simulink model "CSK_Std_PulseTrain"  (R2014b)
settings: Solver=ode23s  StartTime=0.0  StopTime=150  RelTol=1e-12
undefined symbols (not defined in the file or in its folder): Rho, Sigma, x01, x02, x03
settings Model: Creator=Dan  LastModifiedBy=Dan

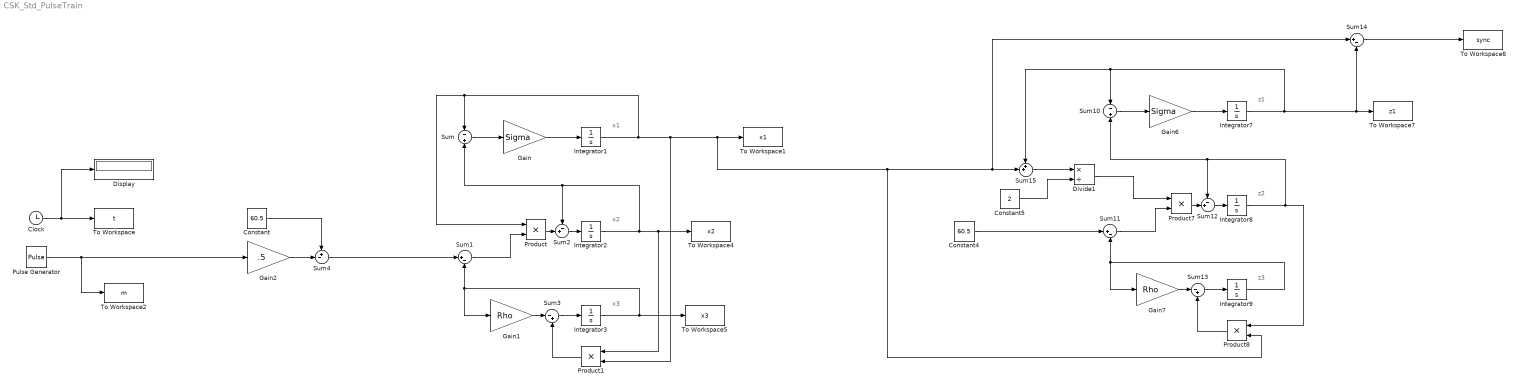
== system CSK_Std_PulseTrain ==
  note: x1
  note: x2
  note: x3
  note: z1
  note: z2
  note: z3
  Clock : Clock
  Constant : Constant  Value=60.5
  Constant4 : Constant  Value=60.5
  Constant5 : Constant  Value=2
  Display : Display
      settings: Decimation=5
  Divide1 : Product  Inputs=*/
  Gain : Gain  Gain=Sigma
  Gain1 : Gain  Gain=Rho
  Gain2 : Gain  Gain=.5
  Gain6 : Gain  Gain=Sigma
  Gain7 : Gain  Gain=Rho
  Integrator1 : Integrator  InitialCondition=x01
  Integrator2 : Integrator  InitialCondition=x02
  Integrator3 : Integrator  InitialCondition=x03
  Integrator7 : Integrator  InitialCondition=x01
  Integrator8 : Integrator  InitialCondition=x02
  Integrator9 : Integrator  InitialCondition=x03
  Product{,1,7..8} (4 alike) : Product
  Pulse Generator : DiscretePulseGenerator  PulseType=Time based  Period=20  PulseWidth=50  PhaseDelay=100
  Sum : Sum  Inputs=-|+
  Sum1 : Sum  Inputs=|+-
  Sum10 : Sum  Inputs=-|+
  Sum11 : Sum  Inputs=|+-
  Sum12 : Sum  Inputs=-+|
  Sum13 : Sum  Inputs=|-+
  Sum14 : Sum  Inputs=|+-
  Sum15 : Sum  Inputs=++|
  Sum2 : Sum  Inputs=-+|
  Sum3 : Sum  Inputs=|-+
  Sum4 : Sum  Inputs=+-|
  To Workspace : ToWorkspace  VariableName=t  SampleTime=-1
  To Workspace1 : ToWorkspace  VariableName=x1  SampleTime=-1
  To Workspace2 : ToWorkspace  VariableName=m  SampleTime=-1
  To Workspace4 : ToWorkspace  VariableName=x2  SampleTime=-1
  To Workspace5 : ToWorkspace  VariableName=x3  SampleTime=-1
  To Workspace6 : ToWorkspace  VariableName=sync  SampleTime=-1
  To Workspace7 : ToWorkspace  VariableName=z1  SampleTime=-1
  wires:
  Gain/1 -> Integrator1/1
  Sum/1 -> Gain/1
  Sum1/1 -> Product/2
  Integrator3/1 -> To Workspace5/1, Gain1/1, Sum1/2
  Sum3/1 -> Integrator3/1
  Product1/1 -> Sum3/2
  Integrator2/1 -> To Workspace4/1, Product1/1, Sum2/1, Sum/2
  Gain1/1 -> Sum3/1
  Gain2/1 -> Sum4/2
  Constant/1 -> Sum4/1
  Sum4/1 -> Sum1/1
  Clock/1 -> Display/1, To Workspace/1
  Product/1 -> Sum2/2
  Sum2/1 -> Integrator2/1
  Pulse Generator/1 -> To Workspace2/1, Gain2/1
  Gain6/1 -> Integrator7/1
  Sum10/1 -> Gain6/1
  Sum11/1 -> Product7/2
  Integrator9/1 -> Gain7/1, Sum11/2
  Sum13/1 -> Integrator9/1
  Product8/1 -> Sum13/2
  Integrator8/1 -> Product8/1, Sum12/1, Sum10/2
  Gain7/1 -> Sum13/1
  Constant4/1 -> Sum11/1
  Product7/1 -> Sum12/2
  Sum12/1 -> Integrator8/1
  Integrator7/1 -> To Workspace7/1, Sum14/2, Sum10/1, Sum15/1
  Integrator1/1 -> Sum/1, Product/1, Product8/2, Sum15/2, Sum14/1, To Workspace1/1, Product1/2
  Sum14/1 -> To Workspace6/1
  Sum15/1 -> Divide1/1
  Divide1/1 -> Product7/1
  Constant5/1 -> Divide1/2
